simulink model "Problem2"  (R2020b)
settings: Solver=VariableStepAuto  StartTime=0.0  StopTime=10.0  RelTol=1e-3
values from neighbouring files (symbols this model uses):
  b = 7    [Prob2.m]
  k1 = 0.6    [Prob2.m]
  k2 = 0.5    [Prob2.m]
  m1 = 5    [Prob2.m]
  m2 = 200    [Prob2.m]
settings Model: Creator=Dell  LastModifiedBy=Dell

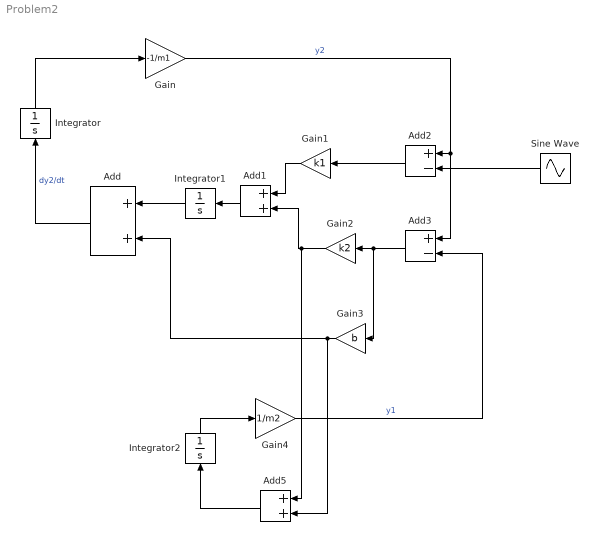
== system Problem2 ==
  Add : Sum
  Add1 : Sum
  Add2 : Sum  Inputs=+-
  Add3 : Sum  Inputs=+-
  Add5 : Sum
  Gain : Gain  Gain=-1/m1
  Gain1 : Gain  Gain=k1
  Gain2 : Gain  Gain=k2
  Gain3 : Gain  Gain=b
  Gain4 : Gain  Gain=1/m2
  Integrator : Integrator
  Integrator1 : Integrator
  Integrator2 : Integrator
  Sine Wave : Sin  Frequency=50  SampleTime=0
  wires:
  Sine Wave/1 -> Add2/2
  Gain1/1 -> Add1/1
  Gain2/1 -> Add5/1, Add1/2
  Add2/1 -> Gain1/1
  Gain/1 -> Add3/1, Add2/1  "y2"
  Add3/1 -> Gain3/1, Gain2/1
  Gain3/1 -> Add5/2, Add/2
  Integrator1/1 -> Add/1
  Add1/1 -> Integrator1/1
  Integrator/1 -> Gain/1
  Add/1 -> Integrator/1  "dy2/dt"
  Integrator2/1 -> Gain4/1
  Add5/1 -> Integrator2/1
  Gain4/1 -> Add3/2  "y1"
